simulink model "untitled1"  (R2024b)
settings: Solver=FixedStepAuto  StartTime=0.0  StopTime=60  FixedStep=0.001  RelTol=1e-3
undefined symbols (not defined in the file): segment_data
settings Model: Creator=lukec  LastModifiedBy=lukec

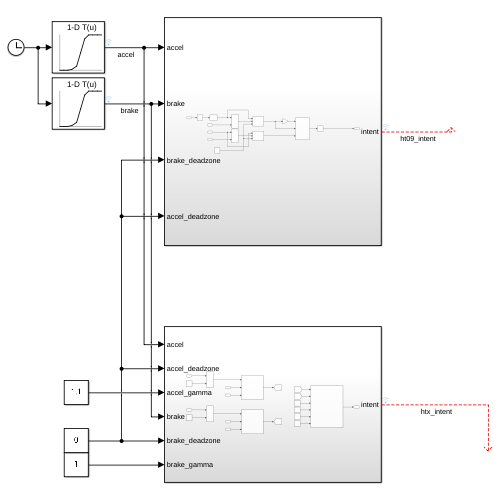
[thumbnail: Simulink's stored preview of the top-level diagram]
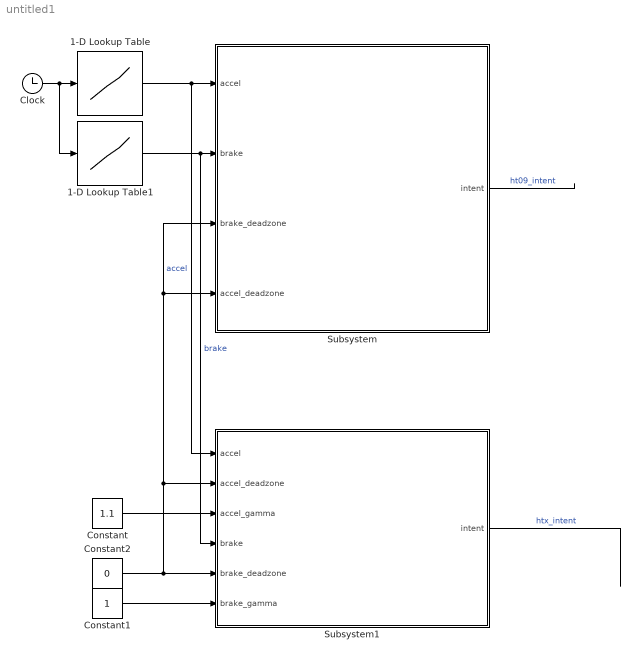
== system untitled1 ==
  1-D Lookup Table : Lookup_n-D  NumberOfTableDimensions=1  BreakpointsForDimension1=segment_data.globalTime  Table=segment_data.pedals_system_data.accel_pedal  ExtrapMethod=Clip  InternalRulePriority=Speed  RndMeth=Simplest
  1-D Lookup Table1 : Lookup_n-D  NumberOfTableDimensions=1  BreakpointsForDimension1=segment_data.globalTime  Table=segment_data.pedals_system_data.brake_pedal  ExtrapMethod=Clip  InternalRulePriority=Speed  RndMeth=Simplest
  Clock : Clock
  Constant : Constant  Value=1.1
  Constant1 : Constant
  Constant2 : Constant  Value=0
  Subsystem : Subsystem
  Subsystem1 : Subsystem
  wires:
  Clock/1 -> 1-D Lookup Table1/1, 1-D Lookup Table/1
  1-D Lookup Table/1 -> Subsystem1/1(accel), Subsystem/1(accel)  "accel"
  1-D Lookup Table1/1 -> Subsystem1/4(brake), Subsystem/2(brake)  "brake"
  Subsystem/1(intent) -> ?  "ht09_intent"
  Constant/1 -> Subsystem1/3(accel_gamma)
  Constant1/1 -> Subsystem1/6(brake_gamma)
  Subsystem1/1(intent) -> ?  "htx_intent"
  Constant2/1 -> Subsystem/3(brake_deadzone), Subsystem/4(accel_deadzone), Subsystem1/2(accel_deadzone), Subsystem1/5(brake_deadzone)

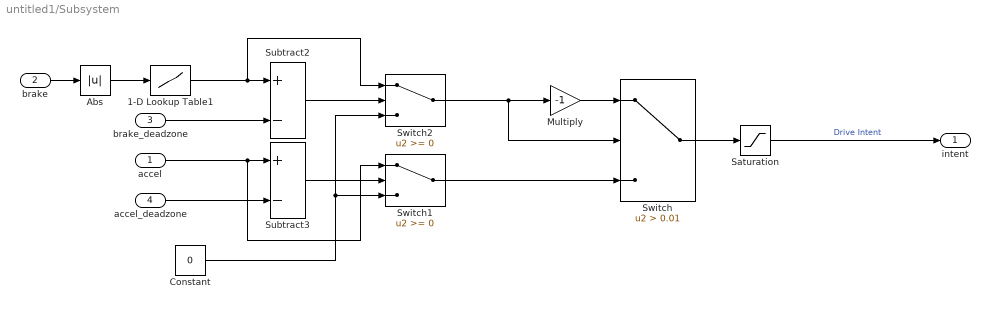
== system untitled1/Subsystem ==
  accel : Inport
  brake : Inport  Port=2
  brake_deadzone : Inport  Port=3
  accel_deadzone : Inport  Port=4
  1-D Lookup Table1 : Lookup_n-D  NumberOfTableDimensions=1  BreakpointsForDimension1=[0 1]  Table=[0 1]  ExtrapMethod=Clip  InternalRulePriority=Speed  RndMeth=Simplest
  Abs : Abs  SaturateOnIntegerOverflow=off
  Constant : Constant  Value=0
  Multiply : Gain  Gain=-1
  Saturation : Saturate  UpperLimit=1  LowerLimit=-1
  Subtract2 : Sum  Inputs=+-
  Subtract3 : Sum  Inputs=+-
  Switch : Switch  Criteria=u2 > Threshold  Threshold=0.01  SaturateOnIntegerOverflow=off  InputSameDT=off
  Switch1 : Switch  SaturateOnIntegerOverflow=off  InputSameDT=off
  Switch2 : Switch  SaturateOnIntegerOverflow=off  InputSameDT=off
  intent : Outport
  wires:
  Abs/1 -> 1-D Lookup Table1/1
  Subtract2/1 -> Switch2/2
  Multiply/1 -> Switch/1
  Saturation/1 -> intent/1  "Drive Intent"
  Switch2/1 -> Switch/2, Multiply/1
  Switch1/1 -> Switch/3
  Subtract3/1 -> Switch1/2
  brake/1 -> Abs/1
  accel_deadzone/1 -> Subtract3/2
  accel/1 -> Switch1/1, Subtract3/1
  brake_deadzone/1 -> Subtract2/2
  1-D Lookup Table1/1 -> Switch2/1, Subtract2/1
  Switch/1 -> Saturation/1
  Constant/1 -> Switch1/3, Switch2/3

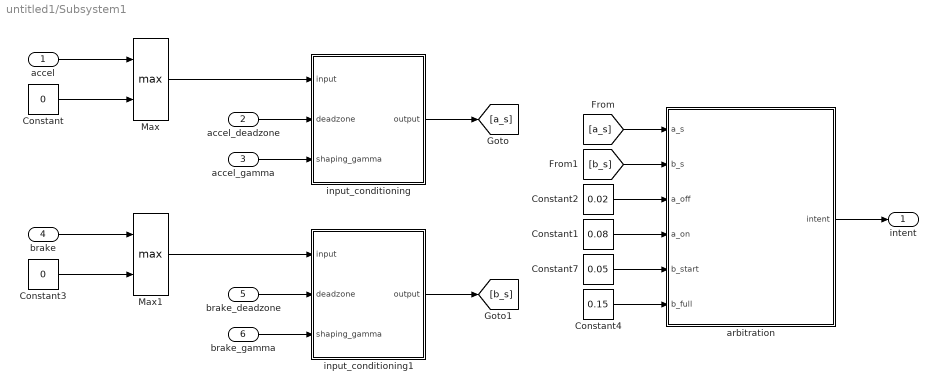
== system untitled1/Subsystem1 ==
  accel : Inport
  accel_deadzone : Inport  Port=2
  accel_gamma : Inport  Port=3
  brake : Inport  Port=4
  brake_deadzone : Inport  Port=5
  brake_gamma : Inport  Port=6
  Constant : Constant  Value=0
  Constant1 : Constant  Value=0.08
  Constant2 : Constant  Value=0.02
  Constant3 : Constant  Value=0
  Constant4 : Constant  Value=0.15
  Constant7 : Constant  Value=0.05
  Max : MinMax  Function=max  Inputs=2
  Max1 : MinMax  Function=max  Inputs=2
  arbitration : Subsystem
  input_conditioning : Subsystem
  input_conditioning1 : Subsystem
  intent : Outport
  wires:
  accel/1 -> Max/1
  Constant/1 -> Max/2
  Max/1 -> input_conditioning/1(input)
  accel_gamma/1 -> input_conditioning/3(shaping_gamma)
  input_conditioning/1(output) -> [a_s]
  accel_deadzone/1 -> input_conditioning/2(deadzone)
  brake/1 -> Max1/1
  Constant3/1 -> Max1/2
  Max1/1 -> input_conditioning1/1(input)
  brake_deadzone/1 -> input_conditioning1/2(deadzone)
  brake_gamma/1 -> input_conditioning1/3(shaping_gamma)
  input_conditioning1/1(output) -> [b_s]
  [a_s] -> arbitration/1(a_s)
  [b_s] -> arbitration/2(b_s)
  Constant7/1 -> arbitration/5(b_start)
  arbitration/1(intent) -> intent/1
  Constant1/1 -> arbitration/4(a_on)
  Constant4/1 -> arbitration/6(b_full)
  Constant2/1 -> arbitration/3(a_off)

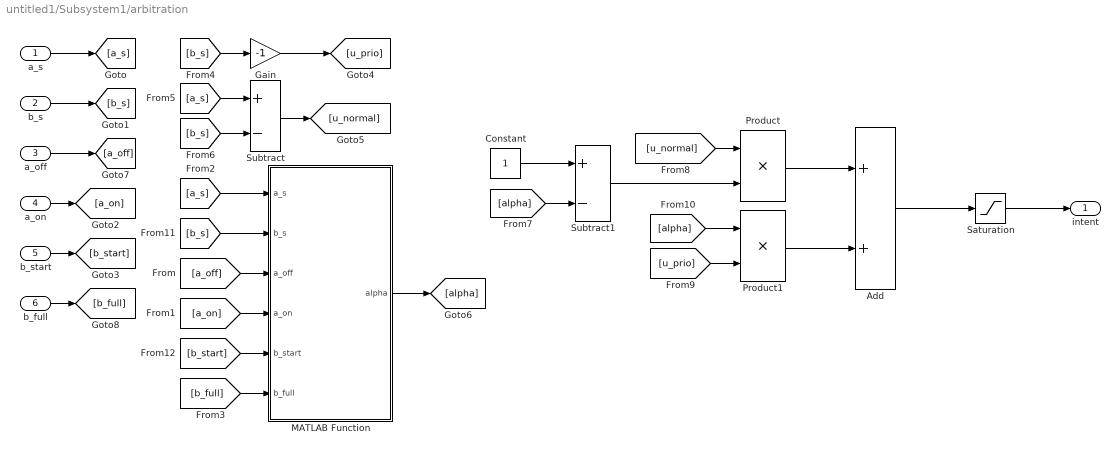
== system untitled1/Subsystem1/arbitration ==
  a_s : Inport
  b_s : Inport  Port=2
  a_off : Inport  Port=3
  a_on : Inport  Port=4
  b_start : Inport  Port=5
  b_full : Inport  Port=6
  Add : Sum
  Constant : Constant
  Gain : Gain  Gain=-1
  MATLAB Function : MATLAB Function  TreatAsAtomicUnit=on
  Product : Product
  Product1 : Product
  Saturation : Saturate  UpperLimit=1  LowerLimit=-1
  Subtract : Sum  Inputs=+-
  Subtract1 : Sum  Inputs=+-
  intent : Outport
  wires:
  a_s/1 -> [a_s]
  b_s/1 -> [b_s]
  b_start/1 -> [b_start]
  [b_s] -> Gain/1
  Gain/1 -> [u_prio]
  [a_s] -> Subtract/1
  [b_s] -> Subtract/2
  Subtract/1 -> [u_normal]
  Saturation/1 -> intent/1
  Constant/1 -> Subtract1/1
  [alpha] -> Subtract1/2
  Subtract1/1 -> Product/2
  [u_normal] -> Product/1
  [u_prio] -> Product1/2
  [alpha] -> Product1/1
  Product/1 -> Add/1
  Product1/1 -> Add/2
  MATLAB Function/1(alpha) -> [alpha]
  Add/1 -> Saturation/1
  a_on/1 -> [a_on]
  b_full/1 -> [b_full]
  [b_s] -> MATLAB Function/2(b_s)
  [a_s] -> MATLAB Function/1(a_s)
  [a_off] -> MATLAB Function/3(a_off)
  [b_start] -> MATLAB Function/5(b_start)
  [b_full] -> MATLAB Function/6(b_full)
  a_off/1 -> [a_off]
  [a_on] -> MATLAB Function/4(a_on)

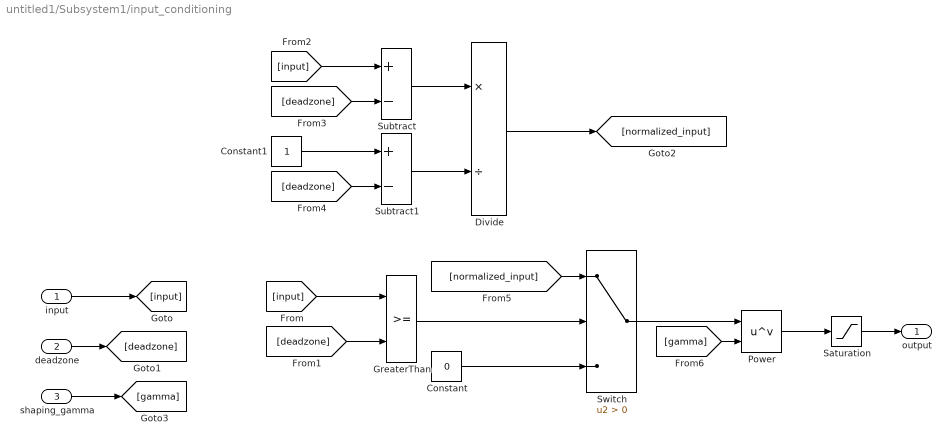
== system untitled1/Subsystem1/input_conditioning ==
  input : Inport
  deadzone : Inport  Port=2
  shaping_gamma : Inport  Port=3
  Constant : Constant  Value=0
  Constant1 : Constant
  Divide : Product  Inputs=*/
  GreaterThan : RelationalOperator  OutDataTypeStr=boolean  RndMeth=Simplest  InputSameDT=off
  Power : Math  Operator=pow
  Saturation : Saturate  UpperLimit=1  LowerLimit=0
  Subtract : Sum  Inputs=+-
  Subtract1 : Sum  Inputs=+-
  Switch : Switch  Criteria=u2 > Threshold  SaturateOnIntegerOverflow=off  InputSameDT=off
  output : Outport
  wires:
  GreaterThan/1 -> Switch/2
  Constant/1 -> Switch/3
  input/1 -> [input]
  deadzone/1 -> [deadzone]
  [input] -> GreaterThan/1
  [deadzone] -> GreaterThan/2
  [input] -> Subtract/1
  [deadzone] -> Subtract/2
  Subtract/1 -> Divide/1
  Constant1/1 -> Subtract1/1
  [deadzone] -> Subtract1/2
  Subtract1/1 -> Divide/2
  Divide/1 -> [normalized_input]
  [normalized_input] -> Switch/1
  shaping_gamma/1 -> [gamma]
  Switch/1 -> Power/1
  [gamma] -> Power/2
  Power/1 -> Saturation/1
  Saturation/1 -> output/1

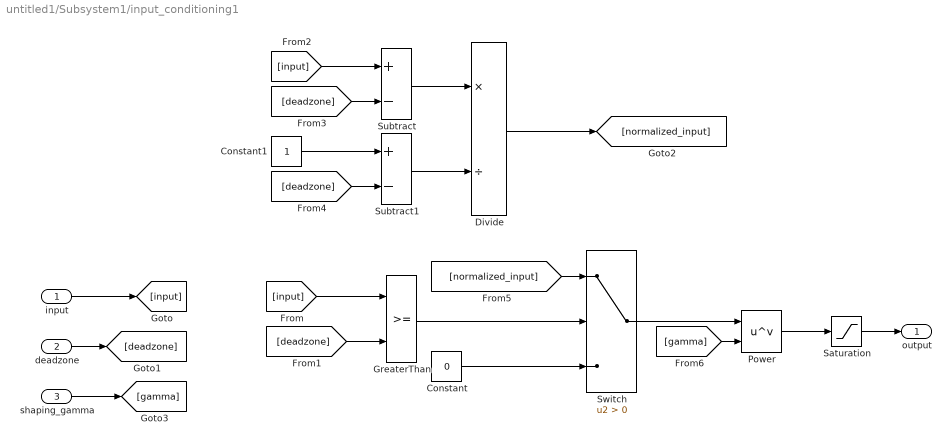
== system untitled1/Subsystem1/input_conditioning1 ==
  input : Inport
  deadzone : Inport  Port=2
  shaping_gamma : Inport  Port=3
  Constant : Constant  Value=0
  Constant1 : Constant
  Divide : Product  Inputs=*/
  GreaterThan : RelationalOperator  OutDataTypeStr=boolean  RndMeth=Simplest  InputSameDT=off
  Power : Math  Operator=pow
  Saturation : Saturate  UpperLimit=1  LowerLimit=0
  Subtract : Sum  Inputs=+-
  Subtract1 : Sum  Inputs=+-
  Switch : Switch  Criteria=u2 > Threshold  SaturateOnIntegerOverflow=off  InputSameDT=off
  output : Outport
  wires:
  Saturation/1 -> output/1
  Power/1 -> Saturation/1
  [gamma] -> Power/2
  Switch/1 -> Power/1
  shaping_gamma/1 -> [gamma]
  [normalized_input] -> Switch/1
  Divide/1 -> [normalized_input]
  Subtract1/1 -> Divide/2
  [deadzone] -> Subtract1/2
  Constant1/1 -> Subtract1/1
  Subtract/1 -> Divide/1
  [deadzone] -> Subtract/2
  [input] -> Subtract/1
  [deadzone] -> GreaterThan/2
  [input] -> GreaterThan/1
  deadzone/1 -> [deadzone]
  input/1 -> [input]
  Constant/1 -> Switch/3
  GreaterThan/1 -> Switch/2

== matlab function untitled1/Subsystem1/arbitration/MATLAB Function ==
  data: a_s input; b_s input; alpha output; a_off input; a_on input; b_start input; b_full input
function alpha = fcn(a_s, b_s, a_off, a_on, b_start, b_full)

% Brake-based alpha
if b_s <= b_start
    alpha_b = 0;
elseif b_s >= b_full
    alpha_b = 1;
else
    alpha_b = (b_s - b_start) / (b_full - b_start);
end

% Smooth throttle gate
if a_s <= a_off
    g = 0;
elseif a_s >= a_on
    g = 1;
else
    g = (a_s - a_off) / (a_on - a_off);
end

alpha = alpha_b * g;
alpha = min(max(alpha,0),1);
